simulink model "Platooning"  (R2014b)
settings: Solver=ode3  SolverMode=SingleTasking  StartTime=0.0  StopTime=300  FixedStep=sampleTimes.main  RelTol=1e-3
PostLoadFcn:
  | initParams
InitFcn:
  | initParams
values from neighbouring files (symbols this model uses):
  data = eval(dataStr)    [TCPReceive.m]    (also in TCPSend.m = reshape(block.InputPort(1).Data, 1, numel(block.InputPort(1))
  spacing = 6    [initParams.m]
undefined symbols (not defined in the file or in its folder): control
libraries: simulink x14
settings Model: Creator=Owen  LastModifiedBy=uos
settings DebuggingCC: SolverPrmCheckMsg=none
settings SFSimCC: SimCustomInitializer=initTORCSLink();  SimCustomTerminator=terminateTORCSLink();  SimUserSources=TORCSLink.c  SimBuildMode=sf_nonincremental_build

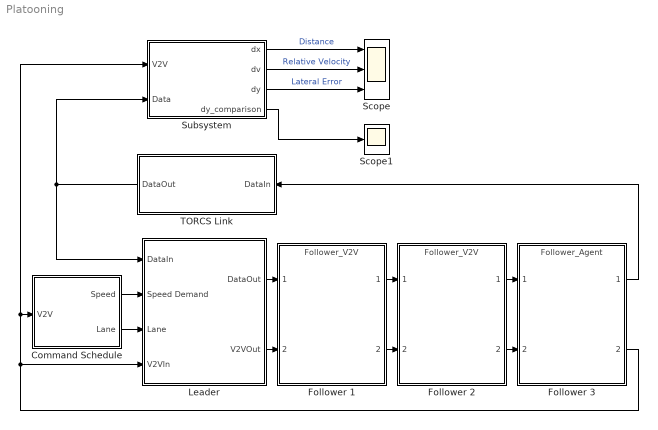
== system Platooning ==
  Command Schedule : Subsystem
  Follower 1 : ModelReference  ModelNameDialog=Follower_V2V.slx  ParameterArgumentNames=vehicle,spacing  ParameterArgumentValues=vehicle,spacing  SimulationMode=Normal  Variant=on  OverrideUsingVariant=varObject1  ModelReferenceVersion=1.970  CopyOfModelName=Follower_V2V.slx  DefaultDataLogging=on  mask{vehicle=2, spacing=spacing}
      mask prompts: spacing "Spacing [m]"
      settings: CopyFcn=|
      | veh = str2num(get_param(gcb, 'vehicle'));
      | veh = veh + 1;
      | set_param(gcb,'vehicle',num2str(veh));
      mask TypeOptions vehicle: 1 | 2 | 3 | 4 | 5 | 6 | 7 | 8 | 9 | 10
  Follower 2 : ModelReference  ModelNameDialog=Follower_V2V.slx  ParameterArgumentNames=vehicle,spacing  ParameterArgumentValues=vehicle,spacing  SimulationMode=Normal  Variant=on  OverrideUsingVariant=varObject1  ModelReferenceVersion=1.970  CopyOfModelName=Follower_V2V.slx  DefaultDataLogging=on  mask{vehicle=3, spacing=spacing}
      mask prompts: spacing "Spacing [m]"
      settings: CopyFcn=|
      | veh = str2num(get_param(gcb, 'vehicle'));
      | veh = veh + 1;
      | set_param(gcb,'vehicle',num2str(veh));
      mask TypeOptions vehicle: 1 | 2 | 3 | 4 | 5 | 6 | 7 | 8 | 9 | 10
  Follower 3 : ModelReference  ModelNameDialog=Follower_Agent.slx  ParameterArgumentNames=vehicle  ParameterArgumentValues=vehicle  SimulationMode=Normal  Variant=on  OverrideUsingVariant=varObject1  ModelReferenceVersion=1.1206  CopyOfModelName=Follower_Agent.slx  DefaultDataLogging=on  mask{vehicle=4}
      settings: CopyFcn=|
      | veh = str2num(get_param(gcb, 'vehicle'));
      | veh = veh + 1;
      | set_param(gcb,'vehicle',num2str(veh));
      mask TypeOptions vehicle: 1 | 2 | 3 | 4 | 5 | 6 | 7 | 8 | 9 | 10
  Leader : Subsystem
  Scope : Scope  NumInputPorts=3
      settings: TimeRange=30  YMin=0~-5~-3  YMax=2000~15~1  SaveName=Errors
  Scope1 : Scope
      settings: TimeRange=30  YMin=-0.5  YMax=2  SaveName=LateralError
  Subsystem : Subsystem
  TORCS Link : Subsystem  LoadFcn=|  InitFcn=|
      LoadFcn=|
      | load VehicleBusses.mat;
      | src = 'TORCSLink.c';
      | init = 'initTORCSLink();';
      | term = 'terminateTORCSLink();';
      | simSrc = get_param(gcs,'SimUserSources');
      | simInit = get_param(gcs,'SimCustomInitializer');
      | simTerm = get_param(gcs,'SimCustomTerminator');
      | 
      | if isempty(strfind(simSrc,src))
      |   fprintf('Adding %s to Custom Sources\n', src);
      |   set_param(gcs,'SimUserSources', [simSrc 10 src]);
      | end
      | 
      | if isempty(strfind(simInit,init))
      |   fprintf('Adding %s to Custom Initialisation Code\n', init);
      |   set_param(gcs,'SimCustomInitializer', [simInit 10 init]);
      | end
      | 
      | if isempty(strfind(simTerm,term))
      |   fprintf('Adding %s to Custom Termination Code\n', term);
      |   set_param(gcs,'SimCustomTerminator', [simTerm 10 term]);
      | end
      | 
      | if isunix
      |     libs = 'librt.so';
      |     simLibs = get_param(gcs,'SimUserLibraries');
      | 
      |     if isempty(strfind(simLibs,libs))
      |       fprintf('Adding %s to Custom Libraries\n', libs);
      |       set_param(gcs,'SimUserLibraries', [simLibs 10 libs]);
      |     end
      | else
      |    set_param(gcs,'SimUserLibraries', '');
      | end
      | 
      | clear src init term simSrc simInit simTerm libs simLibs;
      InitFcn=|
      | load VehicleBusses.mat;
      | src = 'TORCSLink.c';
      | init = 'initTORCSLink();';
      | term = 'terminateTORCSLink();';
      | simSrc = get_param(gcs,'SimUserSources');
      | simInit = get_param(gcs,'SimCustomInitializer');
      | simTerm = get_param(gcs,'SimCustomTerminator');
      | 
      | if isempty(strfind(simSrc,src))
      |   fprintf('Adding %s to Custom Sources\n', src);
      |   set_param(gcs,'SimUserSources', [simSrc 10 src]);
      | end
      | 
      | if isempty(strfind(simInit,init))
      |   fprintf('Adding %s to Custom Initialisation Code\n', init);
      |   set_param(gcs,'SimCustomInitializer', [simInit 10 init]);
      | end
      | 
      | if isempty(strfind(simTerm,term))
      |   fprintf('Adding %s to Custom Termination Code\n', term);
      |   set_param(gcs,'SimCustomTerminator', [simTerm 10 term]);
      | end
      | 
      | if isunix
      |     libs = 'librt.so';
      |     simLibs = get_param(gcs,'SimUserLibraries');
      | 
      |     if isempty(strfind(simLibs,libs))
      |       fprintf('Adding %s to Custom Libraries\n', libs);
      |       set_param(gcs,'SimUserLibraries', [simLibs 10 libs]);
      |     end
      | else
      |    set_param(gcs,'SimUserLibraries', '');
      | end
      | 
      | clear src init term simSrc simInit simTerm libs simLibs;
  wires:
  TORCS Link/1(DataOut) -> Subsystem/2(Data), Leader/1(DataIn)
  Leader/1(DataOut) -> Follower 1/1
  Command Schedule/1(Speed) -> Leader/2(Speed Demand)
  Subsystem/1(dx) -> Scope/1  "Distance"
  Subsystem/2(dv) -> Scope/2  "Relative Velocity"
  Leader/2(V2VOut) -> Follower 1/2
  Follower 1/2 -> Follower 2/2
  Follower 2/1 -> Follower 3/1
  Follower 2/2 -> Follower 3/2
  Subsystem/3(dy) -> Scope/3  "Lateral Error"
  Follower 1/1 -> Follower 2/1
  Command Schedule/2(Lane) -> Leader/3(Lane)
  Subsystem/4(dy_comparison) -> Scope1/1
  Follower 3/1 -> TORCS Link/1(DataIn)
  Follower 3/2 -> Leader/4(V2VIn), Subsystem/1(V2V), Command Schedule/1(V2V)

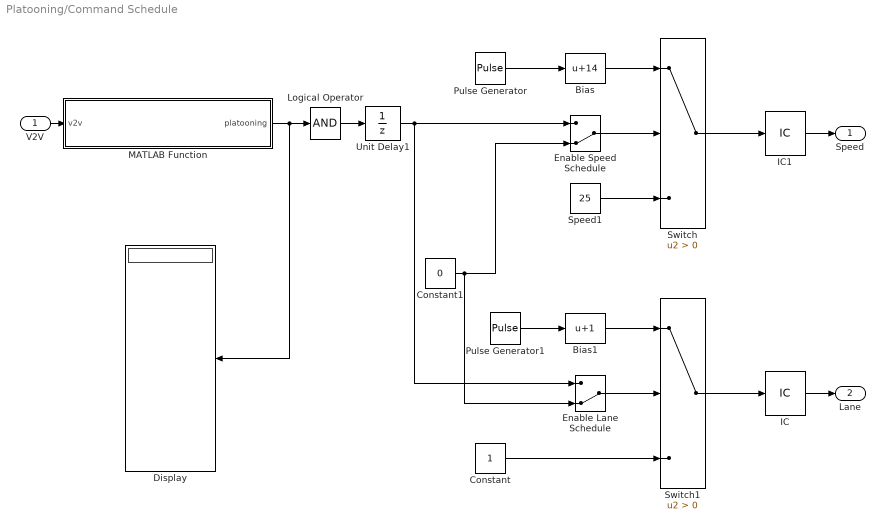
== system Platooning/Command Schedule ==
  V2V : Inport
  Bias : Bias  Bias=14
  Bias1 : Bias  Bias=1
  Constant : Constant
  Constant1 : Constant  Value=0  OutDataTypeStr=boolean
  Display : Display
  Enable Lane Schedule : ManualSwitch  CurrentSetting=0
  Enable Speed Schedule : ManualSwitch  CurrentSetting=0
  IC : InitialCondition
  IC1 : InitialCondition  Value=14
  Logical Operator : Logic  Inputs=1  AllPortsSameDT=off  OutDataTypeStr=boolean
  MATLAB Function : MATLAB Function  TreatAsAtomicUnit=on
  Pulse Generator : DiscretePulseGenerator  PulseType=Time based  Amplitude=11  Period=60  PulseWidth=50  PhaseDelay=33
  Pulse Generator1 : DiscretePulseGenerator  PulseType=Time based  Period=120  PulseWidth=50
  Speed1 : Constant  Value=25
  Switch : Switch  Criteria=u2 > Threshold
  Switch1 : Switch  Criteria=u2 > Threshold
  Unit Delay1 : UnitDelay  SampleTime=-1
  Speed : Outport
  Lane : Outport  Port=2
  wires:
  Pulse Generator/1 -> Bias/1
  Bias/1 -> Switch/1
  Switch/1 -> IC1/1
  Constant/1 -> Switch1/3
  Switch1/1 -> IC/1
  Pulse Generator1/1 -> Bias1/1
  V2V/1 -> MATLAB Function/1(v2v)
  Speed1/1 -> Switch/3
  Bias1/1 -> Switch1/1
  Enable Speed Schedule/1 -> Switch/2
  Enable Lane Schedule/1 -> Switch1/2
  IC/1 -> Lane/1
  IC1/1 -> Speed/1
  MATLAB Function/1(platooning) -> Logical Operator/1, Display/1
  Logical Operator/1 -> Unit Delay1/1
  Constant1/1 -> Enable Speed Schedule/2, Enable Lane Schedule/2
  Unit Delay1/1 -> Enable Speed Schedule/1, Enable Lane Schedule/1

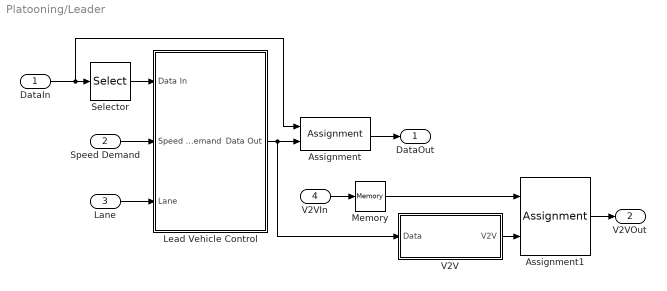
== system Platooning/Leader ==
  DataIn : Inport
  Speed Demand : Inport  Port=2
  Lane : Inport  Port=3
  V2VIn : Inport  Port=4  OutDataTypeStr=Bus: V2VBus  PortDimensions=10
  Assignment : Assignment  DiagnosticForDimensions=Warning
  Assignment1 : Assignment  DiagnosticForDimensions=Warning
  Lead Vehicle Control : Subsystem
  Memory : Memory
  Selector : Selector  InputPortWidth=10
  V2V : Subsystem
  DataOut : Outport
  V2VOut : Outport  Port=2  PortDimensions=10
  wires:
  Speed Demand/1 -> Lead Vehicle Control/2(Speed Demand)
  Lane/1 -> Lead Vehicle Control/3(Lane)
  DataIn/1 -> Assignment/1, Selector/1
  Selector/1 -> Lead Vehicle Control/1(Data In)
  Assignment/1 -> DataOut/1
  Lead Vehicle Control/1(Data Out) -> V2V/1(Data), Assignment/2
  V2V/1(V2V) -> Assignment1/2
  V2VIn/1 -> Memory/1
  Assignment1/1 -> V2VOut/1
  Memory/1 -> Assignment1/1

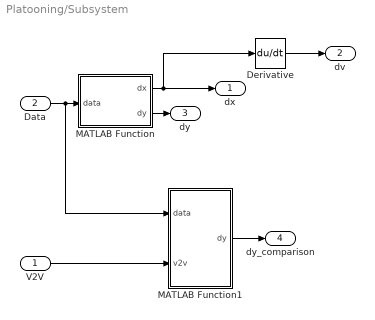
== system Platooning/Subsystem ==
  V2V : Inport
  Data : Inport  Port=2
  Derivative : Derivative
  MATLAB Function : MATLAB Function  TreatAsAtomicUnit=on
  MATLAB Function1 : MATLAB Function  TreatAsAtomicUnit=on
  dx : Outport
  dv : Outport  Port=2
  dy : Outport  Port=3
  dy_comparison : Outport  Port=4
  wires:
  Data/1 -> MATLAB Function1/1(data), MATLAB Function/1(data)
  MATLAB Function/1(dx) -> Derivative/1, dx/1
  Derivative/1 -> dv/1
  MATLAB Function/2(dy) -> dy/1
  V2V/1 -> MATLAB Function1/2(v2v)
  MATLAB Function1/1(dy) -> dy_comparison/1

== system Platooning/TORCS Link ==
  note: This subsystem handles the communicatrion with TORCS via a MATLAB function.
      | The simulation must be configured to run at a fixed sample time equal to the rate at which TORCS updates its robots (0.02s by default)
      | Data returned from TORCS is passed through a First-Order-Hold to allow continuous design in Simulink
      | Data for a maximum of 10 vehicles is returned, but not all vehicles need be present in the race
  DataIn : Inport
  FOHs : Subsystem  TreatAsAtomicUnit=on
  Memory : Memory
  Stop Simulation : Stop
  TORCSLink : MATLAB Function  TreatAsAtomicUnit=on
  DataOut : Outport
  wires:
  Memory/1 -> TORCSLink/1(vehicleDataIn)
  TORCSLink/1(vehicleDataOut) -> FOHs/1(In1)
  FOHs/1(Out1) -> DataOut/1
  DataIn/1 -> Memory/1
  TORCSLink/2(stop) -> Stop Simulation/1

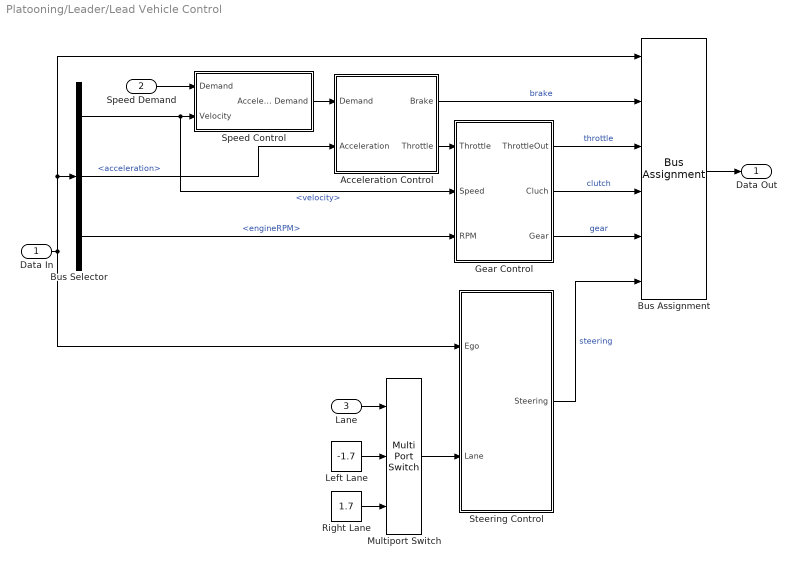
== system Platooning/Leader/Lead Vehicle Control ==
  Data In : Inport
  Speed Demand : Inport  Port=2
  Lane : Inport  Port=3
  Acceleration Control : Subsystem
  Bus Assignment : BusAssignment  AssignedSignals=control.brake,control.throttle,control.clutch,control.gear,control.steering
  Bus Selector : BusSelector  OutputSignals=data.velocity,data.acceleration,data.engineRPM
  Gear Control : Subsystem
  Left Lane : Constant  Value=-1.7
  Multiport Switch : MultiPortSwitch  Inputs=2
  Right Lane : Constant  Value=1.7
  Speed Control : Subsystem
  Steering Control : Subsystem
  Data Out : Outport
  wires:
  Acceleration Control/2(Throttle) -> Gear Control/1(Throttle)
  Data In/1 -> Bus Assignment/1, Bus Selector/1, Steering Control/1(Ego)
  Bus Selector/3 -> Gear Control/3(RPM)  "<engineRPM>"
  Acceleration Control/1(Brake) -> Bus Assignment/2  "brake"
  Gear Control/1(ThrottleOut) -> Bus Assignment/3  "throttle"
  Gear Control/2(Cluch) -> Bus Assignment/4  "clutch"
  Gear Control/3(Gear) -> Bus Assignment/5  "gear"
  Steering Control/1(Steering) -> Bus Assignment/6  "steering"
  Bus Selector/2 -> Acceleration Control/2(Acceleration)  "<acceleration>"
  Speed Control/1(Acceleration Demand) -> Acceleration Control/1(Demand)
  Speed Demand/1 -> Speed Control/1(Demand)
  Multiport Switch/1 -> Steering Control/2(Lane)
  Left Lane/1 -> Multiport Switch/2
  Right Lane/1 -> Multiport Switch/3
  Lane/1 -> Multiport Switch/1
  Bus Selector/1 -> Speed Control/2(Velocity), Gear Control/2(Speed)  "<velocity>"
  Bus Assignment/1 -> Data Out/1

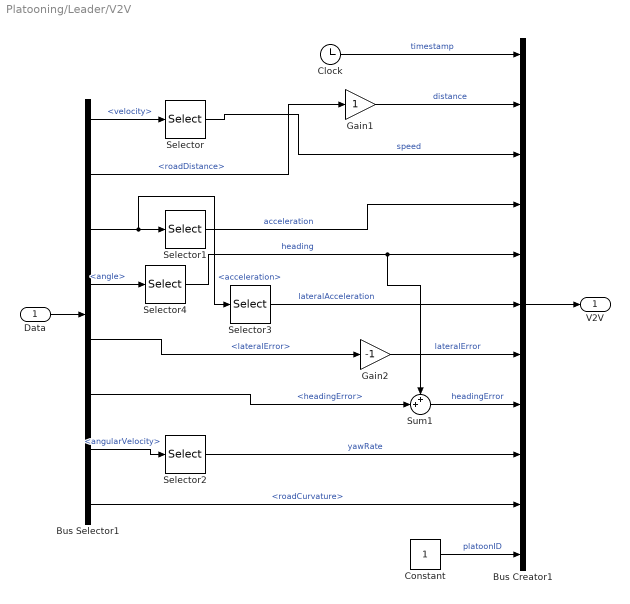
== system Platooning/Leader/V2V ==
  Data : Inport
  Bus Creator1 : BusCreator  Inputs=11  OutDataTypeStr=Bus: V2VBus  NonVirtualBus=on
  Bus Selector1 : BusSelector  OutputSignals=data.velocity,data.roadDistance,data.acceleration,data.angle,data.lateralError,data.headingError,data.angularVelocity,data.roadCurvature
  Clock : Clock
  Constant : Constant  OutDataTypeStr=int32
  Gain1 : Gain
  Gain2 : Gain  Gain=-1
  Selector : Selector  InputPortWidth=3
  Selector1 : Selector  InputPortWidth=3
  Selector2 : Selector  InputPortWidth=3  Indices=3
  Selector3 : Selector  InputPortWidth=3  Indices=2
  Selector4 : Selector  InputPortWidth=3  Indices=3
  Sum1 : Sum  Inputs=++|
  V2V : Outport
  wires:
  Selector1/1 -> Bus Creator1/4  "acceleration"
  Bus Selector1/3 -> Selector3/1, Selector1/1  "<acceleration>"
  Bus Selector1/2 -> Gain1/1  "<roadDistance>"
  Selector/1 -> Bus Creator1/3  "speed"
  Bus Selector1/1 -> Selector/1  "<velocity>"
  Data/1 -> Bus Selector1/1
  Bus Creator1/1 -> V2V/1
  Bus Selector1/6 -> Sum1/2  "<headingError>"
  Bus Selector1/7 -> Selector2/1  "<angularVelocity>"
  Bus Selector1/8 -> Bus Creator1/10  "<roadCurvature>"
  Selector2/1 -> Bus Creator1/9  "yawRate"
  Selector3/1 -> Bus Creator1/6  "lateralAcceleration"
  Bus Selector1/4 -> Selector4/1  "<angle>"
  Selector4/1 -> Bus Creator1/5, Sum1/1  "heading"
  Sum1/1 -> Bus Creator1/8  "headingError"
  Gain1/1 -> Bus Creator1/2  "distance"
  Constant/1 -> Bus Creator1/11  "platoonID"
  Bus Selector1/5 -> Gain2/1  "<lateralError>"
  Gain2/1 -> Bus Creator1/7  "lateralError"
  Clock/1 -> Bus Creator1/1  "timestamp"

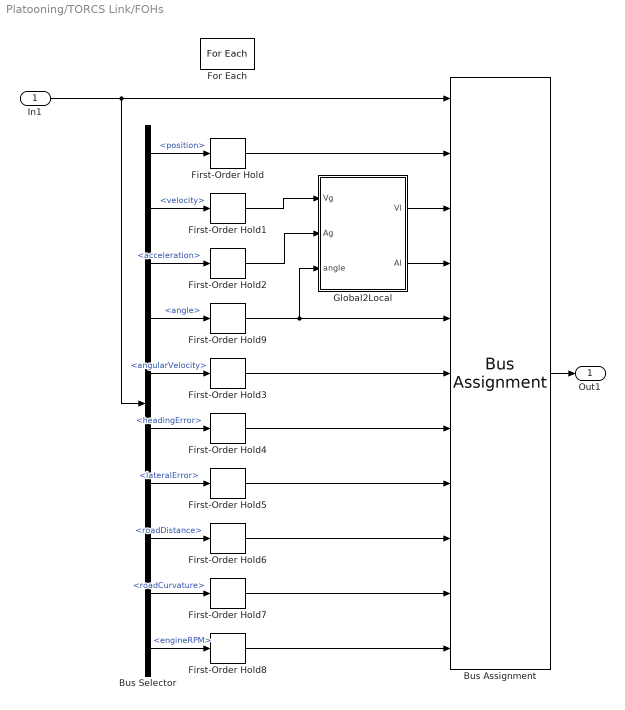
== system Platooning/TORCS Link/FOHs ==
  In1 : Inport  Partition=on  PartitionDimension=1  PartitionWidth=1
  Bus Assignment : BusAssignment  AssignedSignals=data.position,data.velocity,data.acceleration,data.angle,data.angularVelocity,data.headingError,data.lateralError,data.roadDistance,data.roadCurvature,data.engineRPM
  Bus Selector : BusSelector  OutputSignals=data.position,data.velocity,data.acceleration,data.angle,data.angularVelocity,data.headingError,data.lateralError,data.roadDistance,data.roadCurvature,data.engineRPM
  First-Order Hold{,1..9} (10 alike) : simulink/Discrete/First-Order Hold  DisableCoverage=on  Ts=0.02
  For Each : ForEach  DisableCoverage=on  IndexMode=One-based
  Global2Local : MATLAB Function  TreatAsAtomicUnit=on
  Out1 : Outport  ConcatenationDimension=1
  wires:
  Bus Assignment/1 -> Out1/1
  Bus Selector/10 -> First-Order Hold8/1  "<engineRPM>"
  Bus Selector/9 -> First-Order Hold7/1  "<roadCurvature>"
  Bus Selector/8 -> First-Order Hold6/1  "<roadDistance>"
  Bus Selector/7 -> First-Order Hold5/1  "<lateralError>"
  Bus Selector/6 -> First-Order Hold4/1  "<headingError>"
  Bus Selector/5 -> First-Order Hold3/1  "<angularVelocity>"
  Bus Selector/3 -> First-Order Hold2/1  "<acceleration>"
  Bus Selector/2 -> First-Order Hold1/1  "<velocity>"
  Bus Selector/1 -> First-Order Hold/1  "<position>"
  In1/1 -> Bus Assignment/1, Bus Selector/1
  Bus Selector/4 -> First-Order Hold9/1  "<angle>"
  First-Order Hold9/1 -> Global2Local/3(angle), Bus Assignment/5
  First-Order Hold3/1 -> Bus Assignment/6
  First-Order Hold4/1 -> Bus Assignment/7
  First-Order Hold5/1 -> Bus Assignment/8
  First-Order Hold6/1 -> Bus Assignment/9
  First-Order Hold7/1 -> Bus Assignment/10
  First-Order Hold8/1 -> Bus Assignment/11
  First-Order Hold1/1 -> Global2Local/1(Vg)
  First-Order Hold2/1 -> Global2Local/2(Ag)
  First-Order Hold/1 -> Bus Assignment/2
  Global2Local/2(Al) -> Bus Assignment/4
  Global2Local/1(Vl) -> Bus Assignment/3

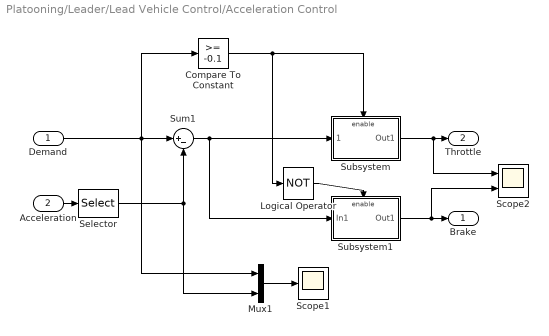
== system Platooning/Leader/Lead Vehicle Control/Acceleration Control ==
  Demand : Inport
  Acceleration : Inport  Port=2
  Compare To Constant : simulink/Logic and Bit Operations/Compare To Constant  relop=>=  const=-0.1  OutDataTypeStr=boolean
  Logical Operator : Logic  Operator=NOT  AllPortsSameDT=off  OutDataTypeStr=boolean
  Mux1 : Mux  Inputs=2
  Scope1 : Scope
      settings: YMax=1  SaveName=ScopeData4
  Scope2 : Scope  NumInputPorts=2
      settings: YMin=-0~-1  YMax=2~1  SaveName=ScopeData6
  Selector : Selector  InputPortWidth=3
  Subsystem : Subsystem
  Subsystem1 : Subsystem
  Sum1 : Sum  Inputs=|+-
  Brake : Outport
  Throttle : Outport  Port=2
  wires:
  Demand/1 -> Compare To Constant/1, Mux1/1, Sum1/1
  Sum1/1 -> Subsystem/1(Demand), Subsystem1/1(In1)
  Subsystem1/1(Out1) -> Scope2/2, Brake/1
  Mux1/1 -> Scope1/1
  Subsystem/1(Out1) -> Scope2/1, Throttle/1
  Compare To Constant/1 -> Subsystem/Enable, Logical Operator/1
  Logical Operator/1 -> Subsystem1/Enable
  Acceleration/1 -> Selector/1
  Selector/1 -> Sum1/2, Mux1/2

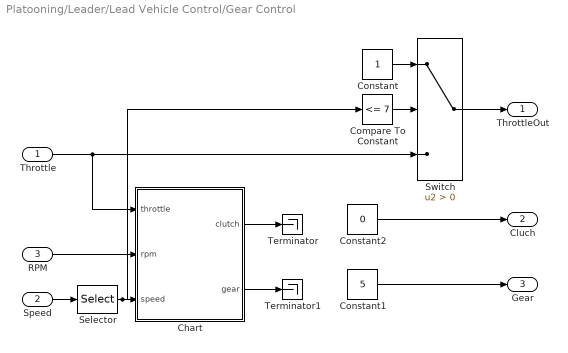
== system Platooning/Leader/Lead Vehicle Control/Gear Control ==
  Throttle : Inport
  Speed : Inport  Port=2
  RPM : Inport  Port=3
  Chart : Stateflow chart  TreatAsAtomicUnit=on
  Compare To Constant : simulink/Logic and Bit Operations/Compare To Constant  relop=<=  const=7  OutDataTypeStr=boolean
  Constant : Constant  OutDataTypeStr=single
  Constant1 : Constant  Value=5  OutDataTypeStr=int32
  Constant2 : Constant  Value=0  OutDataTypeStr=double
  Selector : Selector  InputPortWidth=3
  Switch : Switch  Criteria=u2 > Threshold
  Terminator : Terminator
  Terminator1 : Terminator
  ThrottleOut : Outport
  Cluch : Outport  Port=2
  Gear : Outport  Port=3
  wires:
  Constant2/1 -> Cluch/1
  Constant1/1 -> Gear/1
  Switch/1 -> ThrottleOut/1
  Constant/1 -> Switch/1
  RPM/1 -> Chart/2(rpm)
  Throttle/1 -> Chart/1(throttle), Switch/3
  Speed/1 -> Selector/1
  Selector/1 -> Compare To Constant/1, Chart/3(speed)
  Compare To Constant/1 -> Switch/2
  Chart/1(clutch) -> Terminator/1
  Chart/2(gear) -> Terminator1/1

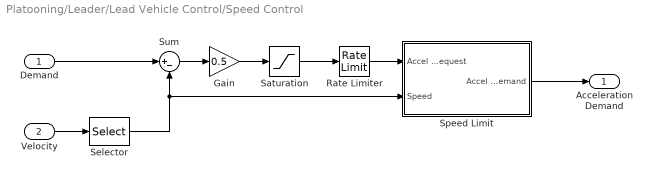
== system Platooning/Leader/Lead Vehicle Control/Speed Control ==
  Demand : Inport
  Velocity : Inport  Port=2
  Gain : Gain  Gain=0.5
  Rate Limiter : RateLimiter  RisingSlewLimit=inf  FallingSlewLimit=-inf  SampleTimeMode=inherited
  Saturation : Saturate  UpperLimit=2  LowerLimit=-4
  Selector : Selector  InputPortWidth=3
  Speed Limit : Subsystem
  Sum : Sum  Inputs=|+-
  Acceleration Demand : Outport
  wires:
  Gain/1 -> Saturation/1
  Sum/1 -> Gain/1
  Demand/1 -> Sum/1
  Velocity/1 -> Selector/1
  Saturation/1 -> Rate Limiter/1
  Selector/1 -> Speed Limit/2(Speed), Sum/2
  Rate Limiter/1 -> Speed Limit/1(Accel Request)
  Speed Limit/1(Accel Demand) -> Acceleration Demand/1

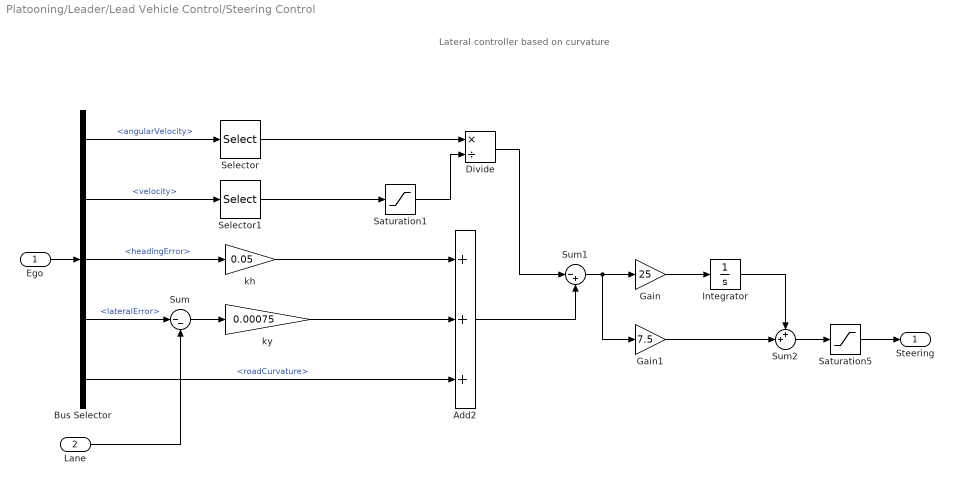
== system Platooning/Leader/Lead Vehicle Control/Steering Control ==
  note: Lateral controller based on curvature
  Ego : Inport
  Lane : Inport  Port=2
  Add2 : Sum  Inputs=+++
  Bus Selector : BusSelector  OutputSignals=data.angularVelocity,data.velocity,data.headingError,data.lateralError,data.roadCurvature
  Divide : Product  Inputs=*/
  Gain : Gain  Gain=25
  Gain1 : Gain  Gain=7.5
  Integrator : Integrator
  Saturation1 : Saturate  UpperLimit=inf  LowerLimit=1
  Saturation5 : Saturate
  Selector : Selector  InputPortWidth=3  Indices=3
  Selector1 : Selector  InputPortWidth=3
  Sum : Sum  Inputs=|--
  Sum1 : Sum  Inputs=|-+
  Sum2 : Sum  Inputs=++|
  kh : Gain  Gain=0.05
  ky : Gain  Gain=0.00075
  Steering : Outport
  wires:
  Ego/1 -> Bus Selector/1
  Bus Selector/1 -> Selector/1  "<angularVelocity>"
  Selector/1 -> Divide/1
  Bus Selector/3 -> kh/1  "<headingError>"
  Bus Selector/4 -> Sum/1  "<lateralError>"
  Lane/1 -> Sum/2
  Sum/1 -> ky/1
  kh/1 -> Add2/1
  ky/1 -> Add2/2
  Bus Selector/5 -> Add2/3  "<roadCurvature>"
  Divide/1 -> Sum1/1
  Bus Selector/2 -> Selector1/1  "<velocity>"
  Selector1/1 -> Saturation1/1
  Saturation5/1 -> Steering/1
  Sum2/1 -> Saturation5/1
  Add2/1 -> Sum1/2
  Gain/1 -> Integrator/1
  Sum1/1 -> Gain/1, Gain1/1
  Gain1/1 -> Sum2/2
  Integrator/1 -> Sum2/1
  Saturation1/1 -> Divide/2

== system Platooning/Leader/Lead Vehicle Control/Acceleration Control/Subsystem ==
  Demand : Inport
  Enable : EnablePort  StatesWhenEnabling=reset
  Gain2 : Gain  Gain=0.5
  Gain4 : Gain  Gain=5
  Integrator : Integrator  LimitOutput=on  UpperSaturationLimit=1  LowerSaturationLimit=-1
  Saturation2 : Saturate  UpperLimit=1  LowerLimit=0
  Sum1 : Sum  Inputs=++|
  Out1 : Outport  OutputWhenDisabled=reset  InitialOutput=0
  wires:
  Demand/1 -> Gain2/1, Gain4/1
  Saturation2/1 -> Out1/1
  Gain2/1 -> Sum1/2
  Integrator/1 -> Sum1/1
  Sum1/1 -> Saturation2/1
  Gain4/1 -> Integrator/1

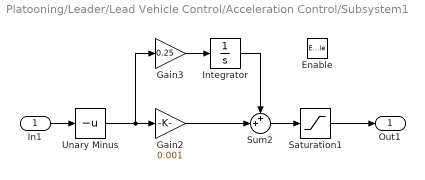
== system Platooning/Leader/Lead Vehicle Control/Acceleration Control/Subsystem1 ==
  In1 : Inport
  Enable : EnablePort  StatesWhenEnabling=reset
  Gain2 : Gain  Gain=0.001
  Gain3 : Gain  Gain=0.25
  Integrator : Integrator  LimitOutput=on  UpperSaturationLimit=1  LowerSaturationLimit=-1
  Saturation1 : Saturate  UpperLimit=1  LowerLimit=0
  Sum2 : Sum  Inputs=++|
  Unary Minus : UnaryMinus
  Out1 : Outport  OutputWhenDisabled=reset  InitialOutput=0
  wires:
  Saturation1/1 -> Out1/1
  Sum2/1 -> Saturation1/1
  In1/1 -> Unary Minus/1
  Gain2/1 -> Sum2/2
  Integrator/1 -> Sum2/1
  Gain3/1 -> Integrator/1
  Unary Minus/1 -> Gain2/1, Gain3/1

== system Platooning/Leader/Lead Vehicle Control/Speed Control/Speed Limit ==
  Accel Request : Inport
  Speed : Inport  Port=2
  70mph : simulink/Logic and Bit Operations/Compare To Constant  relop=<  const=31.3  OutDataTypeStr=boolean
  Compare To Zero : simulink/Logic and Bit Operations/Compare To Zero  relop=<  OutDataTypeStr=boolean
  Constant3 : Constant  Value=0
  Logical Operator : Logic  Operator=OR  AllPortsSameDT=off  OutDataTypeStr=boolean
  Switch : Switch  Criteria=u2 > Threshold
  Accel Demand : Outport
  wires:
  Speed/1 -> 70mph/1
  Compare To Zero/1 -> Logical Operator/1
  Logical Operator/1 -> Switch/2
  70mph/1 -> Logical Operator/2
  Constant3/1 -> Switch/3
  Accel Request/1 -> Compare To Zero/1, Switch/1
  Switch/1 -> Accel Demand/1

== matlab function Platooning/TORCS Link/FOHs/Global2Local ==
  data: Vg input; Ag input; angle input; Vl output; Al output
function [Vl,Al] = fcn(Vg,Ag,angle)
%#codegen

phi=angle(3);
R = [cos(phi) sin(phi) 0; -sin(phi) cos(phi) 0; 0 0 1];

Vl = R*Vg;
Al = R*Ag;

== matlab function Platooning/Subsystem/MATLAB Function ==
  data: data input; dx output; dy output
function [dx, dy] = fcn(data)
%#codegen

N = 4;

dx = zeros(N-1,1);
dy = zeros(N-1,1);

for i=2:N
    X1 = data(i-1).data.position(1:2);
    X2 = data(i).data.position(1:2);
    dx(i-1) = sqrt(sum((X1-X2).^2))-5;
    dy(i-1) = data(i).data.lateralError - data(i-1).data.lateralError;
end

== stateflow chart Platooning/Leader/Lead Vehicle Control/Gear Control/Chart ==
  state ShiftLogic [parallel]
    en: gear = int32(1); minRPM = 2000; maxRPM = 6000;
    settings: executionOrder=1
    state Downshift
      en:clutch = 1;
      ex: gear = gear - int32(1);
    state SteadyState
      en: clutch =0;
    state Upshift
      en: clutch = 1;
      ex: gear = gear + int32(1);
    state Cruise
      en: clutch = 1;
      ex: gear = int32(5);
    (default) -> SteadyState
    SteadyState -> Upshift [order 2] : after(100,msec)[gear < 5 && (rpm > maxRPM || (throttle < 0.25 && rpm > minRPM))]
    SteadyState -> Downshift [order 3] : after(100,msec)[speed < 15 && throttle > 0.25 && (gear > 1 && rpm < minRPM)]
    Upshift -> SteadyState : after(100,msec)
    Downshift -> SteadyState : after(100,msec)
    Cruise -> SteadyState : after(100,msec)
    SteadyState -> Cruise [order 1] : [gear ~=5 && speed > 15]
  data: throttle input; rpm input; clutch output double; minRPM local; maxRPM local; gear output int32; speed input

== matlab function Platooning/Command Schedule/MATLAB Function ==
  data: v2v input Bus: V2VBus size=10; platooning output
function platooning  = fcn(v2v)
%#codegen

platooning = [false false false false false false false false false false];

for i=1:length(v2v)
    platooning(i) = v2v(i).platoonID>0;
end

== matlab function Platooning/Subsystem/MATLAB Function1 ==
  data: dy output; data input; v2v input
function dy  = fcn(data, v2v)
%#codegen

N = 4;
dy = zeros(N-1,1);

for i=2:N
    dy(i-1) = data(i).data.lateralError + v2v(i).lateralError;
end

== matlab function Platooning/TORCS Link/TORCSLink ==
  data: vehicleDataIn input Bus: VehicleBus size=10; vehicleDataOut output Bus: VehicleBus size=10; stop output
function [vehicleDataOut, stop] = TORCSLink(vehicleDataIn)
%#codegen
stop = 0;
flag = int32(0);

% Simulink doesn't like passing the array of structures to C function (no
% idea why?!), so we have to seperate out the three stages

% Update vehicle control values in TORCS
for i=1:10
    flag = coder.ceval('setVehicleControl', int32(i-1), vehicleDataIn(i).control);
    if (flag < 0)
        fprintf('No connection to TORCS!\n');
        stop = 1;
    end
end

% Tell TORCS it can update (this function hangs until new data is
% available)
flag = coder.ceval('updateTORCS');
if (flag < 0)
    fprintf('No data from TORCS! (%d) \n', flag);
    stop = 1;
end

% Read in new data from TORCS
for i=1:10
    % Can't pass this directly to coder.ref
    data = vehicleDataIn(i).data;
    flag = coder.ceval('getVehicleData', int32(i-1), coder.ref(data));
    vehicleDataIn(i).data = data;
    if (flag < 0)
        fprintf('No connection to TORCS!\n');
        stop = 1;
    end
end

vehicleDataOut = vehicleDataIn;
